simulink model "komorek_raka"  (R2024b)
settings: Solver=VariableStepAuto  StartTime=0.0  StopTime=120  RelTol=1e-3
settings Model: Creator=msztu223  LastModifiedBy=msztu223

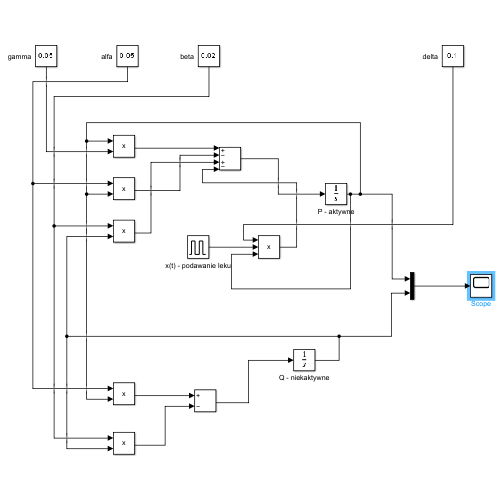
[thumbnail: Simulink's stored preview of the top-level diagram]
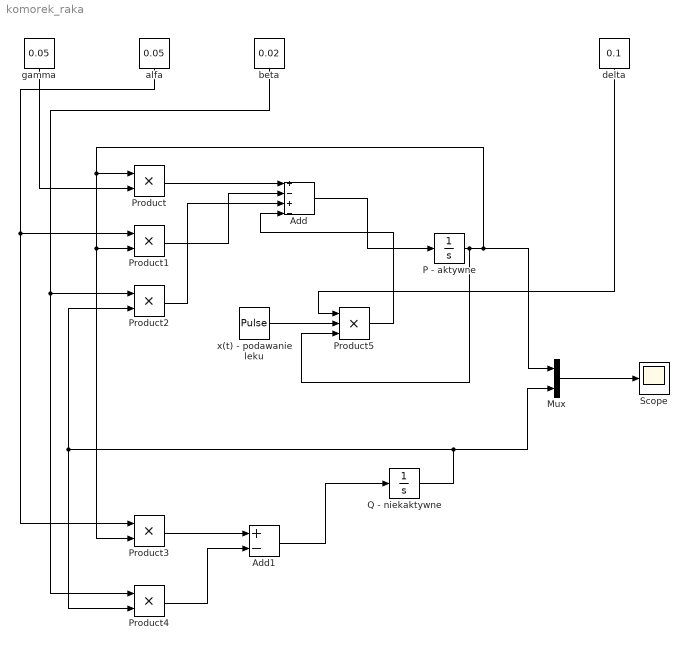
== system komorek_raka ==
  Add : Sum  Inputs=+-+-
  Add1 : Sum  Inputs=+-
  Mux : Mux  Inputs=2
  P - aktywne : Integrator  InitialCondition=100
  Product{,1..4} (5 alike) : Product
  Product5 : Product  Inputs=3
  Q - niekaktywne : Integrator  InitialCondition=50
  Scope : Scope
  alfa : Constant  Value=0.05
  beta : Constant  Value=0.02
  delta : Constant  Value=0.1
  gamma : Constant  Value=0.05
  x(t) - podawanie leku : DiscretePulseGenerator  PulseType=Time based  Amplitude=5  Period=0.1  PulseWidth=15  PhaseDelay=10
  wires:
  P - aktywne/1 -> Product5/3, Mux/1, Product3/2, Product1/2, Product/1
  gamma/1 -> Product/2
  Add/1 -> P - aktywne/1
  alfa/1 -> Product3/1, Product1/1
  Q - niekaktywne/1 -> Mux/2, Product4/2, Product2/2
  beta/1 -> Product4/1, Product2/1
  Product/1 -> Add/1
  Product1/1 -> Add/2
  Product2/1 -> Add/3
  delta/1 -> Product5/1
  x(t) - podawanie leku/1 -> Product5/2
  Product3/1 -> Add1/1
  Product4/1 -> Add1/2
  Add1/1 -> Q - niekaktywne/1
  Mux/1 -> Scope/1
  Product5/1 -> Add/4
